simulink model "PID_Controller"  (R2020a)
settings: Solver=VariableStepAuto  StartTime=0.0  StopTime=100  RelTol=1e-3
PreLoadFcn:
  | m = 1000;
  | b = 50;
  | u = 500;
values from neighbouring files (symbols this model uses):
  Kd = -0.0152524604    [Dictionary_Problem3.sldd]
  Ki = 0.087984779779    [Dictionary_Problem3.sldd]
  Kp = 0.669524552    [Dictionary_Problem3.sldd]
settings Model: DataDictionary=Dictionary_Problem3.sldd  Creator=Admin  LastModifiedBy=Admin
settings DataIOCC: SaveOutput=off  SaveTime=off

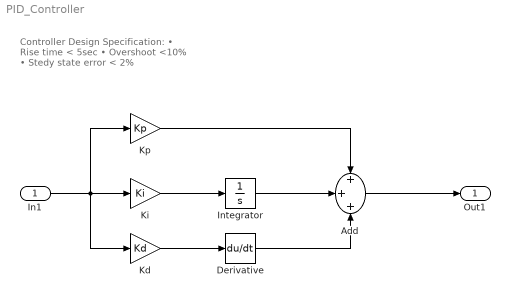
== system PID_Controller ==
  note: Controller Design Specification:
      | • Rise time < 5sec
      | • Overshoot <10%
      | • Stedy state error < 2%
  In1 : Inport  OutDataTypeStr=double  PortDimensions=1  SampleTime=0
  Add : Sum  Inputs=+++
  Derivative : Derivative
  Integrator : Integrator
  Kd : Gain  Gain=Kd
  Ki : Gain  Gain=Ki
  Kp : Gain  Gain=Kp
  Out1 : Outport  OutDataTypeStr=double  PortDimensions=1  SampleTime=0
  wires:
  Kd/1 -> Derivative/1
  Integrator/1 -> Add/2
  Add/1 -> Out1/1
  In1/1 -> Ki/1, Kd/1, Kp/1
  Ki/1 -> Integrator/1
  Kp/1 -> Add/1
  Derivative/1 -> Add/3
